simulink model "vehicle_model_June_25th_2024"  (R2022b)
settings: Solver=ode1  StartTime=0.0  StopTime=1068  FixedStep=0.01  MaxStep=0.1  RelTol=1e-3
values from neighbouring files (symbols this model uses):
  af = 2    [vehicle_load_2024.m]
  cd = 0.30    (= 0.3)    [vehicle_load_2024.m]
  crr = 0.012    [vehicle_load_2024.m]
  mg = mc+mh*np+mp    (= 1870)    [vehicle_load_2024.m]
  n = [0:dn:8000]    [electric_drive_simple.m]
  ro = 1.2041    [vehicle_load_2024.m]
  rt = 4.6    [vehicle_load_2024.m]
  rw = wd/2*25.4e-3+wt*ar/100*1e-3    (= 0.33025)    [vehicle_load_2024.m]
undefined symbols (not defined in the file or in its folder): t_roma_san_basilio, tm, vkm_roma_san_basilio
libraries: simulink x28
settings Model: Creator=claudio.rossi  LastModifiedBy=claudio.rossi
settings DebuggingCC: ParameterOverflowMsg=none  ParameterUnderflowMsg=error  ParameterPrecisionLossMsg=none

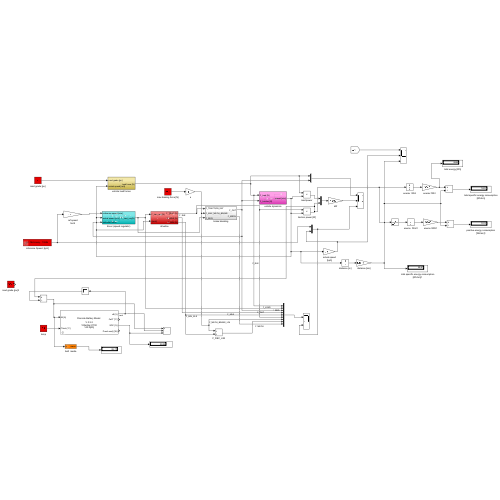
[thumbnail: Simulink's stored preview of the top-level diagram]
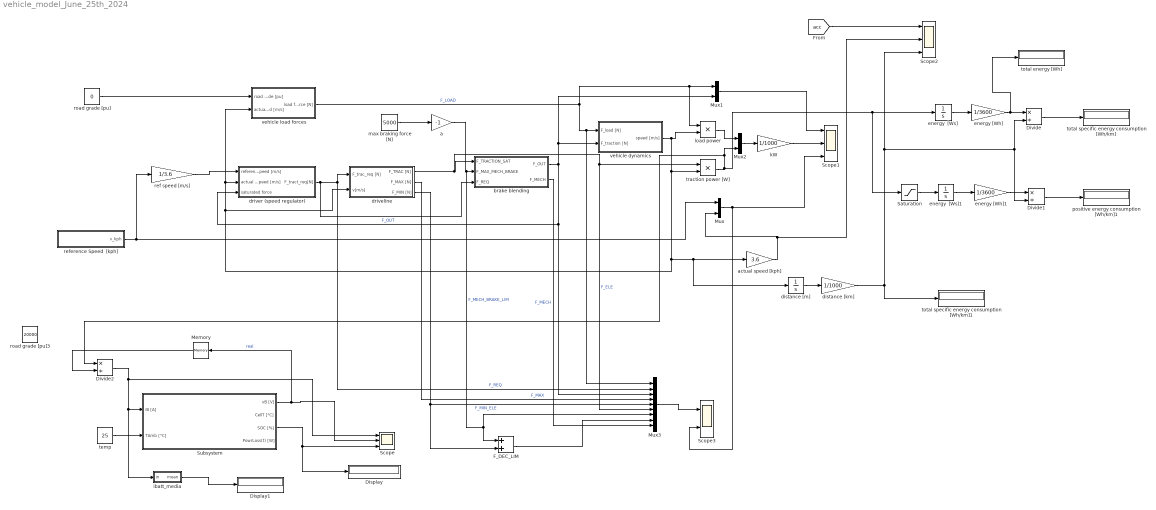
== system vehicle_model_June_25th_2024 ==
  Display : Display
  Display1 : Display
  Divide : Product  Inputs=*/
  Divide1 : Product  Inputs=*/
  Divide2 : Product  Inputs=*/
  F_DEC_LIM : Sum
  Memory : Memory  InitialCondition=400
  Mux : Mux  Inputs=2
  Mux1 : Mux  Inputs=2
  Mux2 : Mux  Inputs=2
  Mux3 : Mux  Inputs=9
  Saturation : Saturate  UpperLimit=inf  LowerLimit=0
  Scope : Scope  NumInputPorts=3
  Scope1 : Scope  NumInputPorts=3
  Scope2 : Scope  NumInputPorts=3
  Scope3 : Scope  NumInputPorts=2
  Subsystem : Subsystem  mask{seriesNumber=100, parallelNumber=28, InitialSOC=100.0, InitialSOH=100.0, BattEff=100.0, CellType=SAMSUNG	21700 	50S	5 [Ah], ThermalModelType=1D With Plastic, ThermReff=off, TRoom=20, R1Therml=2.4, R2Therml=8e-4, R3Therml=9, C1Thermal=62, C2Thermal=4.5}
      mask prompts: seriesNumber "Series Moduels Number [/]"; parallelNumber "Parallel Moduels Number [/]"; InitialSOC "Initial SoC value [%]"; InitialSOH "Initial SoH value [%]"; BattEff "Battery Efficency [%]  (Beta)"; CellType "Cell Type"; ThermalModelType "Thermal Model Type"; ThermReff "Internal Reference"; TRoom "Room Temperautre [°C]"; R1Therml "Core Resistence (R1)  [K/W]"; R2Therml "Can Resistence (R2)  [K/W]"; R3Therml "External Resistence (R3)  [K/W]"; C1Thermal "Core Capacity (C1) [J/K]"; C2Thermal "Can Capacity (C2) [J/K]"
      mask init:
      | if ~exist('batCoeffStudent', 'var')
      |     load('batCoeffStudent.mat')
      | end
      | 
      | switch CellType
      |     case 1 %'IFR18650 EC'
      |         CellNum = 3;
      |     case 2 %'NCR18650 B'
      |         CellNum = 2;
      |     case 3 % NCR18650 GA
      |         CellNum = 4;
      |     case 4 %'INR18650 S'
      |         CellNum = 10;
      |     case 5 %'INR21700 E'
      |         CellNum = 11;
      |     case 6 %'INR21700 S'
      |         CellNum = 12;
      |     case 7 %'INR18650 VTC6'
      |         CellNum = 13;
      |     case 8 %'INR21700 VTC6A'
      |         CellNum = 14;
      |     case 9 % 'INR21700 M50T'
      |         CellNum = 6;
      |     case 10 % 'INR21700 M50T'
      |         CellNum = 5;
      |     case 11 % 'INR21700 P42A'
      |         CellNum = 7;
      |     case 12 % 'INR21700 K42'
      |         CellNum = 8;
      |     case 13 % 'INR21700 K42X'
      |         CellNum = 9;
      | end
      | j = 3;
      | batFormat = batCoeff{CellNum, j};j = j + 1;
      | cellCapacity = batCoeff{CellNum, j};
      | j = 6;
      | voltLim = batCoeff{CellNum, j};j = j + 1;
      | currLim = batCoeff{CellNum, j};
      | j = 8;
      | voc = batCoeff{CellNum, j};j = j + 1;
      | dvoc = batCoeff{CellNum, j};j = j + 1;
      | Cp = batCoeff{CellNum, j};j = j + 1;
      | R0 = batCoeff{CellNum, j};j = j + 1;
      | R0T = batCoeff{CellNum, j};j = j + 1;
      | R0SOH = batCoeff{CellNum, j};j = j + 1;
      | R1 = batCoeff{CellNum, j};j = j + 1;
      | R1T = batCoeff{CellNum, j};j = j + 1;
      | tau1 = batCoeff{CellNum, j};
      mask TypeOptions CellType: OCELL	18650	EC	1.5 [Ah] | PANASONIC	18650	B	3.2 [Ah] | PANASONIC	18650	GA	3.35 [Ah] | SAMSUNG	18650 	35E	3.35 [Ah] | SAMSUNG	21700 	50E	4.9 [Ah] | SAMSUNG	21700 	50S	5 [Ah] | MURATA 	18650	VTC6	3.12 [Ah] | MURATA 	21700	VTC6A	4 [Ah] | LG	21700 	M50T	5 [Ah] | MOLICEL 	21700	M50A	5 [Ah] | MOLICEL	21700	P42A	4.2 [Ah] | KEEPPOWER	21700	K42	4.2 [Ah] | KEEPPOWER	21700	K42X	4.2 [Ah]
      mask TypeOptions ThermalModelType: Constant | 1D With Plastic | 1D No Plastic
      mask DialogControl Container13 Prompt: Pack Parameters
      mask DialogControl Container7 Prompt: Pack Configuration
      mask DialogControl Container14 Prompt: Thermal Parameters
      mask DialogControl Container6 Prompt: Room Temperature
      mask DialogControl Container15 Prompt: Thermal Parameters
      mask Display:
      | fprintf('Discrete Battery Model \n \n \n');
      | fprintf('V 0.3.2');
      | fprintf('\n\n\n %ds%dp %s \n%5.1f[Ah]', seriesNumber,parallelNumber,batFormat, cellCapacity*parallelNumber)
      | 
      | set_param(gcb,'MaskHideContents','off')
  a : Gain  Gain=-1
  actual speed [kph] : Gain  Gain=3.6
  brake blending : Subsystem
  distance [km] : Gain  Gain=1/1000
  distance [m] : Integrator  InitialCondition=0.1
  driveline : Subsystem
  driver (speed regulator) : Subsystem
  energy  [Ws] : Integrator
  energy  [Ws]1 : Integrator
  energy [Wh] : Gain  Gain=1/3600
  energy [Wh]1 : Gain  Gain=1/3600
  ibatt_media : Subsystem  mask{T=1068}
      mask prompts: T "period [s]"
  kW : Gain  Gain=1/1000
  load power : Product
  max braking force [N] : Constant  Value=5000
  positive energy consumption [Wh/km]1 : Display
  ref speed [m/s] : Gain  Gain=1/3.6
  reference Speed  [kph] : Subsystem  mask{slct=Art. Motorway - 1068s}
      mask prompts: slct "Select Cycle"
      mask help: by mtb
      mask init:
      | load('ECE_EUDC_Artemis_Bologna_Roma_WLTC_EE_bus.mat')
      mask TypeOptions slct: ECE15 - 195s | EUDC - 400s | Art. Urban - 994s | Art. Rural - 1083s | Art. Motorway - 1068s | Roma S.Basilio - 522s | BO Viali slow - 1321s | BO Viali quick - 1215s | WLTC city - 1022s | WLTC class1 - 1612s | WLTC class2 - 1800s | WLTC class3a - 1800s | WLTC class3b - 1800s | Bus line BO 27A - 3246s | Bus line BO 27B - 3058s | Bus line BO 33 - 1850s | EE Bike Cycle - 1201s | 130kph
      mask DialogControl DescGroupVar Prompt: LEMAD Speed Cycle
      mask DialogControl DescTextVar Prompt: Function that outputs the speed reference in Km/h for the desired cycle
      mask Display:
      | switch slct
      |     case 1
      |         fprintf('ECE15 - 195s');
      |     case 2
      |         fprintf('EUDC - 400s');
      |     case 3
      |         fprintf('Art. Urban - 994s');
      |     case 4
      |         fprintf('Art. Rural - 1083s');
      |     case 5
      |         fprintf('Art. Motorway - 1068s');
      |     case 6
      |         fprintf('Roma S.Basilio - 522s');
      |     case 7
      |         fprintf('BO Viali slow - 1321s');
      |     case 8
      |         fprintf('BO Viali quick - 1215s');
      |     case 9
      |         fprintf('WLTC city - 1022s');
      |     case 10
      |         fprintf('WLTC class1 - 1612s');
      |     case 11
      |         fprintf('WLTC class2 - 1800s');
      |     case 12
      |         fprintf('WLTC class3a - 1800s');
      |     case 13
      |         fprintf('WLTC class3b - 1800s');
      |     case 14
      |         fprintf('Bus line BO 27A - 3246s');
      |     case 15
      |         fprintf('Bus line BO 27A - 3058s');
      |     case 16
      |         fprintf('Bus line BO 33 - 1850s');
      |     case 17
      |         fprintf('EE Bike Cycle - 1201s');
      |     case 18
      |         fprintf('130kph');
      | end
  road grade [pu] : Constant  Value=0
  road grade [pu]3 : Constant  Value=20000
  temp : Constant  Value=25
  total energy [Wh] : Display
  total specific energy consumption [Wh/km] : Display
  total specific energy consumption [Wh/km]1 : Display
  traction power [W] : Product
  vehicle dynamics : Subsystem
  vehicle load forces : Subsystem
  wires:
  driver (speed regulator)/1(F_tract_req[N]) -> brake blending/3(F_REQ), driveline/1(F_trac_req [N]), Mux3/2  "F_REQ"
  vehicle load forces/1(load force [N]) -> load power/1, Mux1/1, Mux3/1, vehicle dynamics/1(F_load [N])  "F_LOAD"
  road grade [pu]/1 -> vehicle load forces/1(road grade [pu])
  ref speed [m/s]/1 -> driver (speed regulator)/1(reference speed [m/s])
  vehicle dynamics/1(speed [m/s]) -> load power/2, driveline/2(v[m/s]), vehicle load forces/2(actual speed [m/s]), driver (speed regulator)/2(actual speed [m/s]), distance [m]/1, actual speed [kph]/1, traction power [W]/2
  reference Speed  [kph]/1(v_kph) -> Mux/1, ref speed [m/s]/1
  actual speed [kph]/1 -> Scope2/2, Mux/2
  Mux/1 -> Scope3/2, Scope1/3
  load power/1 -> Mux2/1
  traction power [W]/1 -> Divide2/1, Mux2/2, Saturation/1, energy  [Ws]/1
  Mux2/1 -> kW/1
  Mux1/1 -> Scope1/1
  kW/1 -> Scope1/2
  [acc] -> Scope2/1
  distance [m]/1 -> distance [km]/1
  distance [km]/1 -> total specific energy consumption [Wh/km]1/1, Divide1/2, Divide/2, Scope2/3
  energy  [Ws]/1 -> energy [Wh]/1
  energy [Wh]/1 -> total energy [Wh]/1, Divide/1
  Divide/1 -> total specific energy consumption [Wh/km]/1
  Saturation/1 -> energy  [Ws]1/1
  energy  [Ws]1/1 -> energy [Wh]1/1
  energy [Wh]1/1 -> Divide1/1
  Divide1/1 -> positive energy consumption [Wh/km]1/1
  Mux3/1 -> Scope3/1
  driveline/2(F_MAX [N]) -> Mux3/4  "F_MAX"
  driveline/3(F_MIN [N]) -> F_DEC_LIM/2, Mux3/5  "F_MIN_ELE"
  brake blending/1(F_OUT) -> Mux3/3, driver (speed regulator)/3(saturated force), vehicle dynamics/2(F_traction [N]), Mux1/2  "F_OUT"
  driveline/1(F_TRAC [N]) -> traction power [W]/1, Mux3/6, brake blending/1(F_TRACTION_SAT)  "F_ELE"
  max braking force [N]/1 -> a/1
  a/1 -> F_DEC_LIM/1, Mux3/7, brake blending/2(F_MAX_MECH_BRAKE)  "F_MECH_BRAKE_LIM"
  F_DEC_LIM/1 -> Mux3/8
  brake blending/2(F_MECH) -> Mux3/9  "F_MECH"
  Subsystem/1(vB [V]) -> Memory/1, Scope/2  "real"
  Divide2/1 -> Subsystem/1(iB [A]), ibatt_media/1(in), Scope/1
  temp/1 -> Subsystem/2(TAmb [°C])
  Subsystem/3(SOC [%]) -> Display/1, Scope/3
  ibatt_media/1(mean) -> Display1/1
  Memory/1 -> Divide2/2

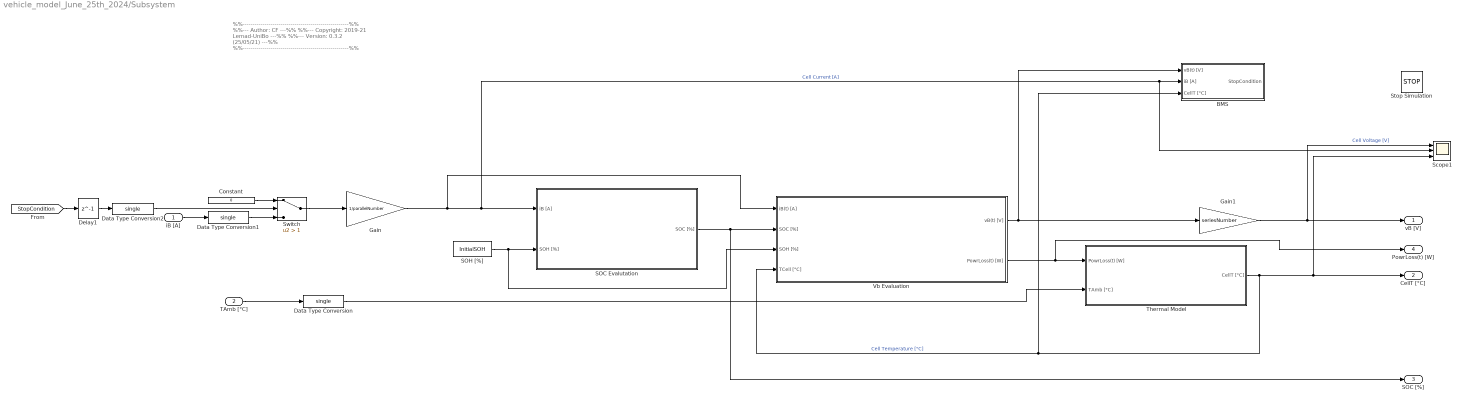
== system vehicle_model_June_25th_2024/Subsystem ==
  note: %%-----------------------------------------------------%%
      | %%--- Author: 	CF 					 ---%%
      | %%--- Copyright: 	2019-21 Lemad-UniBo ---%%
      | %%--- Version:	0.3.2 (25/05/21)		 ---%%
      | %%-----------------------------------------------------%%
  iB [A] : Inport
  TAmb [°C] : Inport  Port=2
  BMS : Subsystem
  Constant : Constant  Value=0  OutDataTypeStr=single
  Data Type Conversion : DataTypeConversion  OutDataTypeStr=single  SaturateOnIntegerOverflow=off  RndMeth=Floor
  Data Type Conversion1 : DataTypeConversion  OutDataTypeStr=single  SaturateOnIntegerOverflow=off  RndMeth=Floor
  Data Type Conversion2 : DataTypeConversion  OutDataTypeStr=single  SaturateOnIntegerOverflow=off  RndMeth=Floor
  Delay1 : Delay  DelayLength=1
  Gain : Gain  Gain=1/parallelNumber  OutDataTypeStr=single
  Gain1 : Gain  Gain=seriesNumber
  SOC Evalutation : Subsystem
      mask Display: image('SOC.PNG'); % Use "Edit Image" on toolstrip to change.
  SOH [%] : Constant  Value=InitialSOH  OutDataTypeStr=single
  Scope1 : Scope  NumInputPorts=3
  Stop Simulation : Stop
  Switch : Switch  Criteria=u2 > Threshold  Threshold=1  SaturateOnIntegerOverflow=off  InputSameDT=off
  Thermal Model : Subsystem
      mask Display: image('ThermModel.png'); % Use "Edit Image" on toolstrip to change.
  Vb Evaluation : Subsystem
      mask Display: image('SP_scheme.PNG'); % Use "Edit Image" on toolstrip to change.
  vB [V] : Outport
  CellT [°C] : Outport  Port=2
  SOC [%] : Outport  Port=3
  PowrLoss(t) [W] : Outport  Port=4
  wires:
  SOH [%]/1 -> Vb Evaluation/3(SOH [%]), SOC Evalutation/2(SOH [%])
  SOC Evalutation/1(SOC [%]) -> SOC [%]/1, Vb Evaluation/2(SOC [%])
  TAmb [°C]/1 -> Data Type Conversion/1
  Gain/1 -> SOC Evalutation/1(iB [A]), Scope1/2, BMS/2(iB [A]), Vb Evaluation/1(iB(t) [A])  "Cell Current [A]"
  Vb Evaluation/1(vB(t) [V]) -> Gain1/1, BMS/1(vB(t) [V])
  Gain1/1 -> Scope1/1, vB [V]/1  "Cell Voltage [V]"
  Vb Evaluation/2(PowrLoss(t) [W]) -> PowrLoss(t) [W]/1, Thermal Model/1(PowrLoss(t) [W])
  Thermal Model/1(CellT [°C]) -> BMS/3(CellT [°C]), Vb Evaluation/4(TCell [°C]), Scope1/3, CellT [°C]/1  "Cell Temperature [°C]"
  Switch/1 -> Gain/1
  iB [A]/1 -> Data Type Conversion1/1
  Constant/1 -> Switch/1
  Delay1/1 -> Data Type Conversion2/1
  [StopCondition] -> Delay1/1
  Data Type Conversion/1 -> Thermal Model/2(TAmb [°C])
  Data Type Conversion1/1 -> Switch/3
  Data Type Conversion2/1 -> Switch/2

== system vehicle_model_June_25th_2024/brake blending ==
  F_TRACTION_SAT : Inport
  F_MAX_MECH_BRAKE : Inport  Port=2
  F_REQ : Inport  Port=3
  Add : Sum
  Constant : Constant  Value=0
  Saturation Dynamic : simulink/Discontinuities/Saturation Dynamic  OutMin=[]  OutMax=[]  OutDataTypeStr=Inherit: Same as second input  OutDataType=fixdt(1, 16)  OutScaling=2^-10  DoSatur=off
  Subtract : Sum  Inputs=+-
  Switch : Switch  Criteria=u2 > Threshold  SaturateOnIntegerOverflow=off  InputSameDT=off
  F_OUT : Outport
  F_MECH : Outport  Port=2
  wires:
  F_TRACTION_SAT/1 -> Add/2, Subtract/2, Switch/1, Switch/2
  Switch/1 -> Subtract/1, F_OUT/1
  F_MAX_MECH_BRAKE/1 -> Add/1
  F_REQ/1 -> Saturation Dynamic/3
  Constant/1 -> Saturation Dynamic/1
  Add/1 -> Saturation Dynamic/2
  Saturation Dynamic/1 -> Switch/3
  Subtract/1 -> F_MECH/1

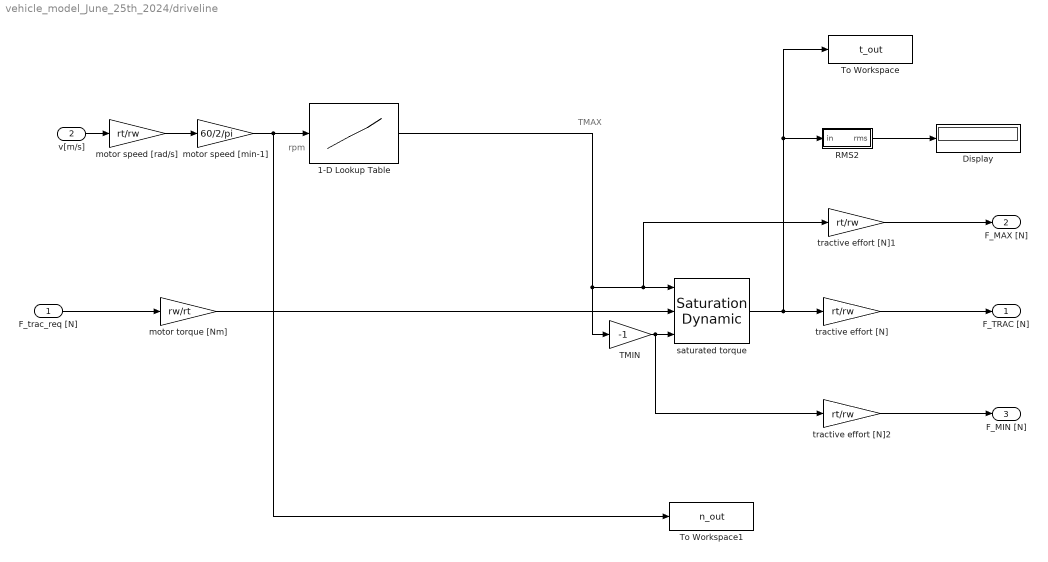
== system vehicle_model_June_25th_2024/driveline ==
  note: rpm
  note: TMAX
  F_trac_req [N] : Inport
  v[m/s] : Inport  Port=2
  1-D Lookup Table : Lookup_n-D  NumberOfTableDimensions=1  BreakpointsForDimension1=n  Table=tm  InternalRulePriority=Speed  RndMeth=Simplest
  Display : Display
  RMS2 : Subsystem  mask{T=1068}
      mask prompts: T "period [s]"
  TMIN : Gain  Gain=-1
  To Workspace : ToWorkspace  VariableName=t_out  SampleTime=-1
  To Workspace1 : ToWorkspace  VariableName=n_out  SampleTime=-1
  motor speed [min-1] : Gain  Gain=60/2/pi
  motor speed [rad/s] : Gain  Gain=rt/rw
  motor torque [Nm] : Gain  Gain=rw/rt
  saturated torque : simulink/Discontinuities/Saturation Dynamic  OutMin=[]  OutMax=[]  OutDataTypeStr=Inherit: Same as second input  OutDataType=fixdt(1, 16)  OutScaling=2^-10  DoSatur=off
  tractive effort [N] : Gain  Gain=rt/rw
  tractive effort [N]1 : Gain  Gain=rt/rw
  tractive effort [N]2 : Gain  Gain=rt/rw
  F_TRAC [N] : Outport
  F_MAX [N] : Outport  Port=2
  F_MIN [N] : Outport  Port=3
  wires:
  v[m/s]/1 -> motor speed [rad/s]/1
  motor speed [rad/s]/1 -> motor speed [min-1]/1
  motor speed [min-1]/1 -> To Workspace1/1, 1-D Lookup Table/1
  F_trac_req [N]/1 -> motor torque [Nm]/1
  1-D Lookup Table/1 -> TMIN/1, tractive effort [N]1/1, saturated torque/1
  TMIN/1 -> tractive effort [N]2/1, saturated torque/3
  motor torque [Nm]/1 -> saturated torque/2
  saturated torque/1 -> To Workspace/1, RMS2/1(in), tractive effort [N]/1
  tractive effort [N]/1 -> F_TRAC [N]/1
  tractive effort [N]1/1 -> F_MAX [N]/1
  tractive effort [N]2/1 -> F_MIN [N]/1
  RMS2/1(rms) -> Display/1

== system vehicle_model_June_25th_2024/driver (speed regulator) ==
  reference speed [m/s] : Inport
  actual speed [m/s] : Inport  Port=2
  saturated force : Inport  Port=3
  Add : Sum
  Integrator : Integrator
  KI : Gain  Gain=5000
  KP : Gain  Gain=15000
  K_desat : Gain  Gain=100
  speed error : Sum  Inputs=+-
  speed error1 : Sum  Inputs=+-
  speed error2 : Sum  Inputs=+-
  F_tract_req[N] : Outport
  wires:
  reference speed [m/s]/1 -> speed error/1
  actual speed [m/s]/1 -> speed error/2
  speed error/1 -> KI/1, KP/1
  KP/1 -> Add/1
  Integrator/1 -> Add/2
  saturated force/1 -> speed error1/2
  speed error2/1 -> Integrator/1
  KI/1 -> speed error2/1
  Add/1 -> speed error1/1, F_tract_req[N]/1
  K_desat/1 -> speed error2/2
  speed error1/1 -> K_desat/1

== system vehicle_model_June_25th_2024/ibatt_media ==
  in : Inport
  Gain1 : Gain  Gain=1/T
  Integrator : Integrator
  Subtract : Sum  Inputs=+-
  Transport Delay : TransportDelay  DelayTime=T  BufferSize=200000
  mean : Outport
  wires:
  Integrator/1 -> Subtract/1, Transport Delay/1
  in/1 -> Integrator/1
  Subtract/1 -> Gain1/1
  Transport Delay/1 -> Subtract/2
  Gain1/1 -> mean/1

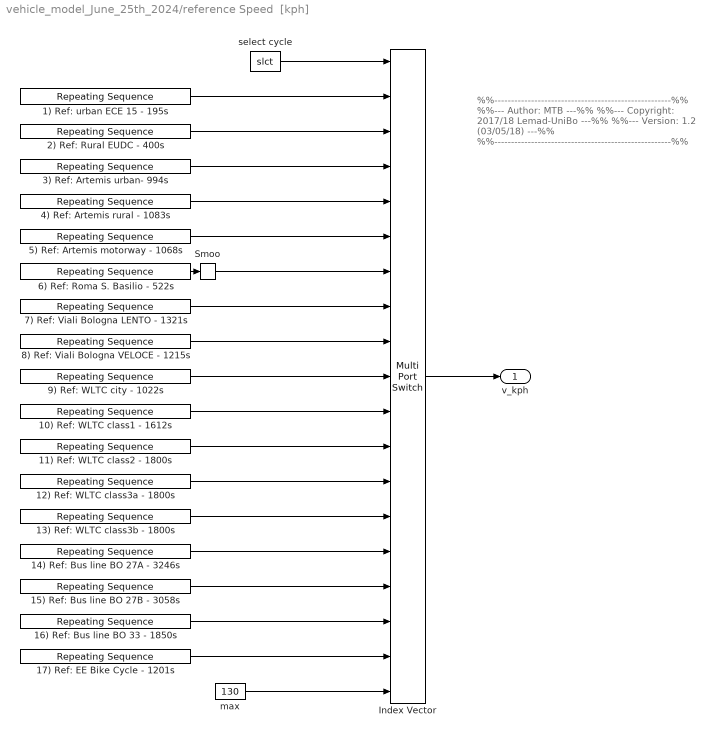
== system vehicle_model_June_25th_2024/reference Speed  [kph] ==
  note: %%-----------------------------------------------------%%
      | %%--- Author: 	MTB 				 ---%%
      | %%--- Copyright: 	2017/18 Lemad-UniBo ---%%
      | %%--- Version:	1.2 (03/05/18)		 ---%%
      | %%-----------------------------------------------------%%
  1) Ref: urban ECE 15 - 195s : simulink/Sources/Repeating Sequence  rep_seq_t=[0 11 15 23 28 49 55 61 85 96 117 123 134 143 155 163 178 188 195]  rep_seq_y=[0 0 15 15 0 0 15 15 32 32 0 0 15 35 50 50 35 35 0]
  10) Ref: WLTC class1 - 1612s : simulink/Sources/Repeating Sequence  rep_seq_t=t_wltc_class_1  rep_seq_y=vkm_wltc_class_1
  11) Ref: WLTC class2 - 1800s : simulink/Sources/Repeating Sequence  rep_seq_t=t_wltc_class_2  rep_seq_y=vkm_wltc_class_2
  12) Ref: WLTC class3a - 1800s : simulink/Sources/Repeating Sequence  rep_seq_t=t_wltc_class_3a  rep_seq_y=vkm_wltc_class_3a
  13) Ref: WLTC class3b - 1800s : simulink/Sources/Repeating Sequence  rep_seq_t=t_wltc_class_3b  rep_seq_y=vkm_wltc_class_3b
  14) Ref: Bus line BO 27A - 3246s : simulink/Sources/Repeating Sequence  rep_seq_t=t_bus_27A  rep_seq_y=vkm_bus_27A
  15) Ref: Bus line BO 27B - 3058s : simulink/Sources/Repeating Sequence  rep_seq_t=t_bus_27B  rep_seq_y=vkm_bus_27B
  16) Ref: Bus line BO 33 - 1850s : simulink/Sources/Repeating Sequence  rep_seq_t=t_bus_33  rep_seq_y=vkm_bus_33
  17) Ref: EE Bike Cycle - 1201s : simulink/Sources/Repeating Sequence  rep_seq_t=EE_time  rep_seq_y=EE_Speedkmh
  2) Ref: Rural EUDC - 400s : simulink/Sources/Repeating Sequence  rep_seq_t=t_eudc  rep_seq_y=vkm_eudc
  3) Ref: Artemis urban- 994s : simulink/Sources/Repeating Sequence  rep_seq_t=t_artemis_urban  rep_seq_y=vkm_artemis_urban
  4) Ref: Artemis rural - 1083s : simulink/Sources/Repeating Sequence  rep_seq_t=t_artemis_rural  rep_seq_y=vkm_artemis_rural
  5) Ref: Artemis motorway - 1068s : simulink/Sources/Repeating Sequence  rep_seq_t=t_artemis_motorway130  rep_seq_y=vkm_artemis_motorway130
  6) Ref: Roma S. Basilio - 522s : simulink/Sources/Repeating Sequence  rep_seq_t=[-0.1 ; t_roma_san_basilio]  rep_seq_y=[0 ; vkm_roma_san_basilio]
  7) Ref: Viali Bologna LENTO - 1321s : simulink/Sources/Repeating Sequence  rep_seq_t=t_bologna_viali_lento  rep_seq_y=vkm_bologna_viali_lento
  8) Ref: Viali Bologna VELOCE - 1215s : simulink/Sources/Repeating Sequence  rep_seq_t=t_bologna_viali_veloce  rep_seq_y=vkm_bologna_viali_veloce
  9) Ref: WLTC city - 1022s : simulink/Sources/Repeating Sequence  rep_seq_t=t_wltc_city  rep_seq_y=vkm_wltc_city
  Index Vector : MultiPortSwitch  Inputs=18  SaturateOnIntegerOverflow=off  InputSameDT=off
  Smoo : RateLimiter  RisingSlewLimit=9  FallingSlewLimit=-9  SampleTimeMode=inherited
  max : Constant  Value=130
  select cycle : Constant  Value=slct
  v_kph : Outport
  wires:
  max/1 -> Index Vector/19
  17) Ref: EE Bike Cycle - 1201s/1 -> Index Vector/18
  16) Ref: Bus line BO 33 - 1850s/1 -> Index Vector/17
  15) Ref: Bus line BO 27B - 3058s/1 -> Index Vector/16
  14) Ref: Bus line BO 27A - 3246s/1 -> Index Vector/15
  select cycle/1 -> Index Vector/1
  2) Ref: Rural EUDC - 400s/1 -> Index Vector/3
  3) Ref: Artemis urban- 994s/1 -> Index Vector/4
  4) Ref: Artemis rural - 1083s/1 -> Index Vector/5
  5) Ref: Artemis motorway - 1068s/1 -> Index Vector/6
  Smoo/1 -> Index Vector/7
  7) Ref: Viali Bologna LENTO - 1321s/1 -> Index Vector/8
  8) Ref: Viali Bologna VELOCE - 1215s/1 -> Index Vector/9
  9) Ref: WLTC city - 1022s/1 -> Index Vector/10
  10) Ref: WLTC class1 - 1612s/1 -> Index Vector/11
  11) Ref: WLTC class2 - 1800s/1 -> Index Vector/12
  12) Ref: WLTC class3a - 1800s/1 -> Index Vector/13
  13) Ref: WLTC class3b - 1800s/1 -> Index Vector/14
  Index Vector/1 -> v_kph/1
  6) Ref: Roma S. Basilio - 522s/1 -> Smoo/1
  1) Ref: urban ECE 15 - 195s/1 -> Index Vector/2

== system vehicle_model_June_25th_2024/vehicle dynamics ==
  F_load [N] : Inport
  F_traction [N] : Inport  Port=2
  Facc [N] : Sum  Inputs=+-
  Integrator : Integrator
  acceleration [m/s^2] : Gain  Gain=1/mg
  speed [m/s] : Outport
  tag scope: acc=global
  wires:
  F_traction [N]/1 -> Facc [N]/1
  F_load [N]/1 -> Facc [N]/2
  Facc [N]/1 -> acceleration [m/s^2]/1
  acceleration [m/s^2]/1 -> [acc], Integrator/1
  Integrator/1 -> speed [m/s]/1

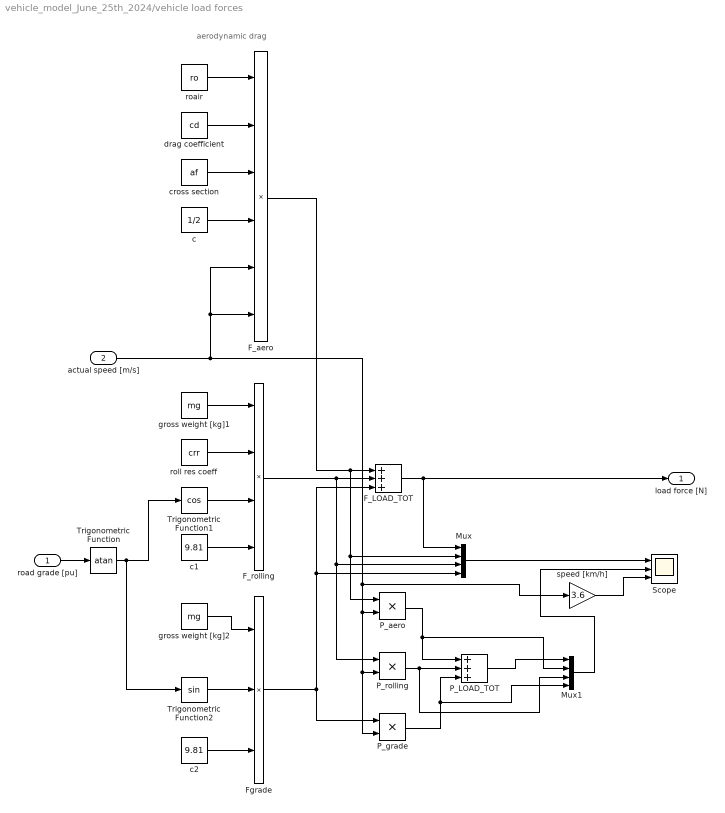
== system vehicle_model_June_25th_2024/vehicle load forces ==
  note: aerodynamic drag
  road grade [pu] : Inport
  actual speed [m/s] : Inport  Port=2
  F_LOAD_TOT : Sum  Inputs=+++
  F_aero : Product  Inputs=6
  F_rolling : Product  Inputs=4
  "Fgrade " : Product  Inputs=3
  Mux : Mux
  Mux1 : Mux
  P_LOAD_TOT : Sum  Inputs=+++
  P_aero : Product
  P_grade : Product
  P_rolling : Product
  Scope : Scope  NumInputPorts=3
  Trigonometric Function : Trigonometry  Operator=atan
  Trigonometric Function1 : Trigonometry  Operator=cos
  Trigonometric Function2 : Trigonometry
  c : Constant  Value=1/2
  c1 : Constant  Value=9.81
  c2 : Constant  Value=9.81
  "cross section " : Constant  Value=af
  drag coefficient : Constant  Value=cd
  gross weight [kg]1 : Constant  Value=mg
  gross weight [kg]2 : Constant  Value=mg
  roair : Constant  Value=ro
  roll res coeff : Constant  Value=crr
  speed [km/h] : Gain  Gain=3.6
  load force [N] : Outport
  wires:
  roair/1 -> F_aero/1
  drag coefficient/1 -> F_aero/2
  "cross section "/1 -> F_aero/3
  c/1 -> F_aero/4
  actual speed [m/s]/1 -> speed [km/h]/1, P_grade/2, P_rolling/2, P_aero/2, F_aero/5, F_aero/6
  road grade [pu]/1 -> Trigonometric Function/1
  gross weight [kg]1/1 -> F_rolling/1
  roll res coeff/1 -> F_rolling/2
  Trigonometric Function1/1 -> F_rolling/3
  c1/1 -> F_rolling/4
  gross weight [kg]2/1 -> "Fgrade "/1
  Trigonometric Function/1 -> Trigonometric Function2/1, Trigonometric Function1/1
  Trigonometric Function2/1 -> "Fgrade "/2
  c2/1 -> "Fgrade "/3
  F_aero/1 -> P_aero/1, Mux/2, F_LOAD_TOT/1
  F_rolling/1 -> P_rolling/1, Mux/3, F_LOAD_TOT/2
  "Fgrade "/1 -> Mux/4, F_LOAD_TOT/3, P_grade/1
  F_LOAD_TOT/1 -> Mux/1, load force [N]/1
  Mux/1 -> Scope/1
  P_aero/1 -> Mux1/2, P_LOAD_TOT/1
  P_rolling/1 -> Mux1/3, P_LOAD_TOT/2
  P_grade/1 -> P_LOAD_TOT/3, Mux1/4
  P_LOAD_TOT/1 -> Mux1/1
  Mux1/1 -> Scope/2
  speed [km/h]/1 -> Scope/3

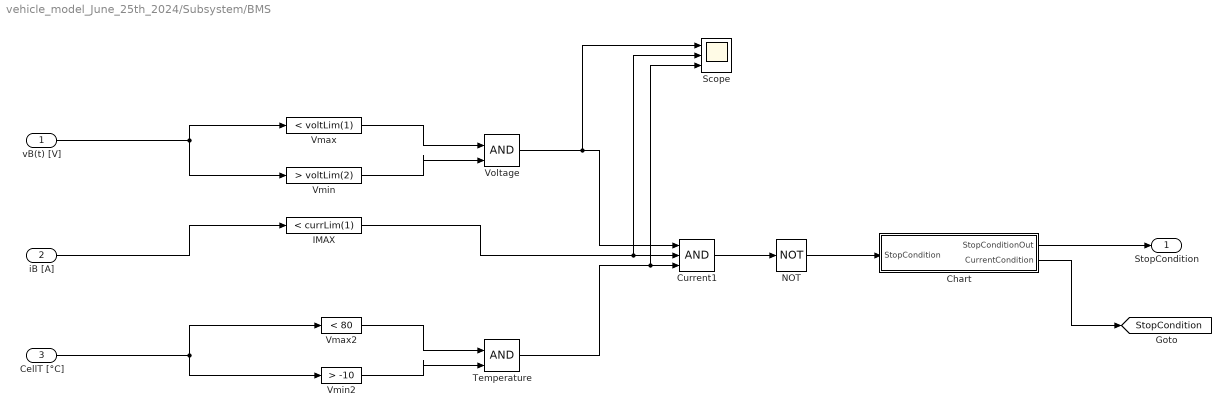
== system vehicle_model_June_25th_2024/Subsystem/BMS ==
  vB(t) [V] : Inport
  iB [A] : Inport  Port=2
  CellT [°C] : Inport  Port=3
  Chart : Stateflow chart  TreatAsAtomicUnit=on
  Current1 : Logic  Inputs=3  IconShape=distinctive  AllPortsSameDT=off  OutDataTypeStr=boolean
  IMAX : simulink/Logic and Bit Operations/Compare To Constant  relop=<  const=currLim(1)  OutDataTypeStr=boolean
  NOT : Logic  Operator=NOT  IconShape=distinctive  AllPortsSameDT=off  OutDataTypeStr=boolean
  Scope : Scope  NumInputPorts=3
  Temperature : Logic  IconShape=distinctive  AllPortsSameDT=off  OutDataTypeStr=boolean
  Vmax : simulink/Logic and Bit Operations/Compare To Constant  relop=<  const=voltLim(1)  OutDataTypeStr=boolean
  Vmax2 : simulink/Logic and Bit Operations/Compare To Constant  relop=<  const=80  OutDataTypeStr=boolean
  Vmin : simulink/Logic and Bit Operations/Compare To Constant  relop=>  const=voltLim(2)  OutDataTypeStr=boolean
  Vmin2 : simulink/Logic and Bit Operations/Compare To Constant  relop=>  const=-10  OutDataTypeStr=boolean
  Voltage : Logic  IconShape=distinctive  AllPortsSameDT=off  OutDataTypeStr=boolean
  StopCondition : Outport
  tag scope: StopCondition=global
  wires:
  Vmin/1 -> Voltage/2
  Vmax/1 -> Voltage/1
  IMAX/1 -> Scope/2, Current1/2
  Voltage/1 -> Scope/1, Current1/1
  Temperature/1 -> Scope/3, Current1/3
  Current1/1 -> NOT/1
  vB(t) [V]/1 -> Vmin/1, Vmax/1
  Vmax2/1 -> Temperature/1
  Vmin2/1 -> Temperature/2
  CellT [°C]/1 -> Vmax2/1, Vmin2/1
  iB [A]/1 -> IMAX/1
  NOT/1 -> Chart/1(StopCondition)
  Chart/2(CurrentCondition) -> [StopCondition]
  Chart/1(StopConditionOut) -> StopCondition/1

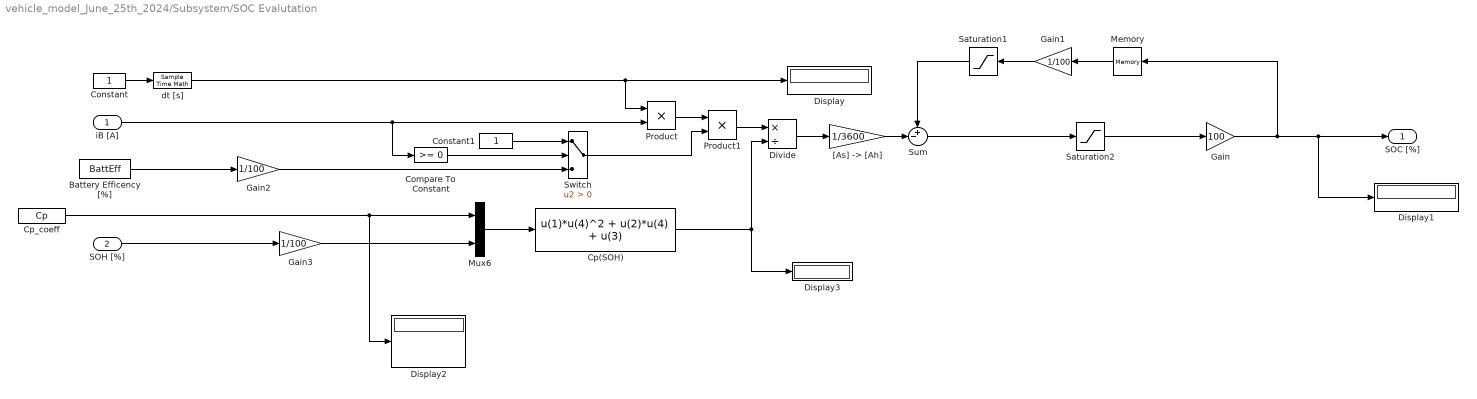
== system vehicle_model_June_25th_2024/Subsystem/SOC Evalutation ==
  iB [A] : Inport
  SOH [%] : Inport  Port=2
  Battery Efficency [%] : Constant  Value=BattEff  OutDataTypeStr=single
  Compare To Constant : simulink/Logic and Bit Operations/Compare To Constant  relop=>=  const=0  OutDataTypeStr=boolean
  Constant : Constant  OutDataTypeStr=single
  Constant1 : Constant  OutDataTypeStr=single
  Cp(SOH) : Fcn  Expr=u(1)*u(4)^2 + u(2)*u(4) + u(3)
  Cp_coeff : Constant  Value=Cp  OutDataTypeStr=single
  Display{,1..3} (4 alike) : Display
  Divide : Product  Inputs=*/
  Gain : Gain  Gain=100
  Gain1 : Gain  Gain=1/100
  Gain2 : Gain  Gain=1/100
  Gain3 : Gain  Gain=1/100
  Memory : Memory  InitialCondition=InitialSOC
  Mux6 : Mux  Inputs=2
  Product : Product  OutDataTypeStr=single
  Product1 : Product
  Saturation1 : Saturate  UpperLimit=0.999  LowerLimit=0.001
  Saturation2 : Saturate  UpperLimit=0.999  LowerLimit=0.001
  Sum : Sum  Inputs=+-|  OutDataTypeStr=single
  Switch : Switch  Criteria=u2 > Threshold  SaturateOnIntegerOverflow=off  InputSameDT=off
  "[As] -> [Ah]" : Gain  Gain=1/3600
  dt [s] : SampleTimeMath  TsampMathOp=Ts Only
  SOC [%] : Outport
  wires:
  Cp_coeff/1 -> Display2/1, Mux6/1
  Mux6/1 -> Cp(SOH)/1
  Constant/1 -> dt [s]/1
  dt [s]/1 -> Display/1, Product/1
  Cp(SOH)/1 -> Display3/1, Divide/2
  Gain/1 -> Memory/1, Display1/1, SOC [%]/1
  Saturation1/1 -> Sum/1
  Sum/1 -> Saturation2/1
  Memory/1 -> Gain1/1
  Gain1/1 -> Saturation1/1
  iB [A]/1 -> Compare To Constant/1, Product/2
  "[As] -> [Ah]"/1 -> Sum/2
  Divide/1 -> "[As] -> [Ah]"/1
  Product1/1 -> Divide/1
  Product/1 -> Product1/1
  Switch/1 -> Product1/2
  Constant1/1 -> Switch/1
  Compare To Constant/1 -> Switch/2
  Battery Efficency [%]/1 -> Gain2/1
  Gain2/1 -> Switch/3
  SOH [%]/1 -> Gain3/1
  Gain3/1 -> Mux6/2
  Saturation2/1 -> Gain/1

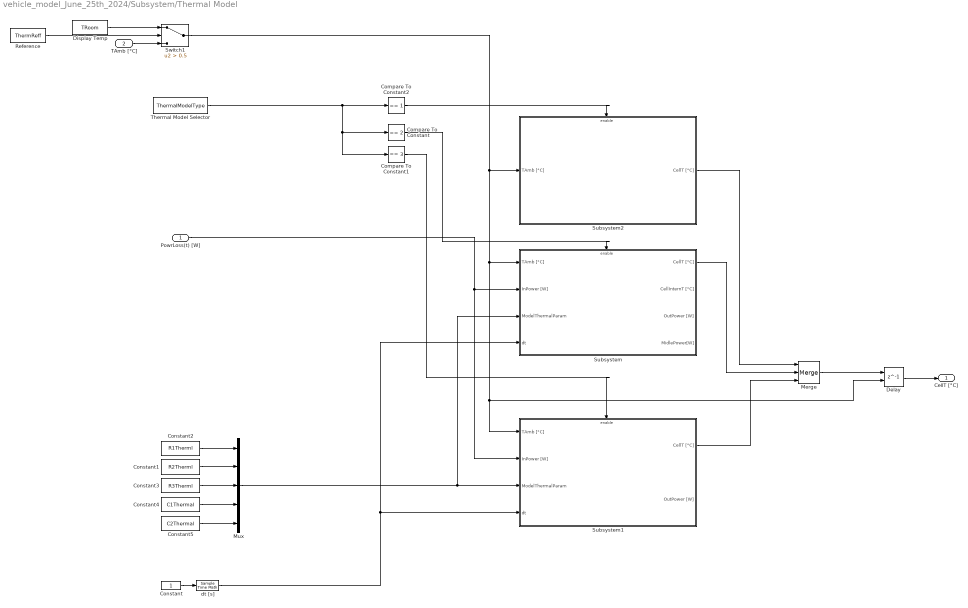
== system vehicle_model_June_25th_2024/Subsystem/Thermal Model ==
  PowrLoss(t) [W] : Inport
  TAmb [°C] : Inport  Port=2
  Compare To Constant : simulink/Logic and Bit Operations/Compare To Constant  relop===  const=2  OutDataTypeStr=boolean
  Compare To Constant1 : simulink/Logic and Bit Operations/Compare To Constant  relop===  const=3  OutDataTypeStr=boolean
  Compare To Constant2 : simulink/Logic and Bit Operations/Compare To Constant  relop===  const=1  OutDataTypeStr=boolean
  Constant : Constant  OutDataTypeStr=single
  Constant1 : Constant  Value=R2Therml  OutDataTypeStr=single
  Constant2 : Constant  Value=R1Therml  OutDataTypeStr=single
  Constant3 : Constant  Value=R3Therml  OutDataTypeStr=single
  Constant4 : Constant  Value=C1Thermal  OutDataTypeStr=single
  Constant5 : Constant  Value=C2Thermal  OutDataTypeStr=single
  Delay : Delay  DelayLength=1  InitialConditionSource=Input port
      settings: InputPortMap=u0,p4
  Display Temp : Constant  Value=TRoom  OutDataTypeStr=single
  Merge : Merge  Inputs=3
  Mux : Mux  Inputs=5
  Reference : Constant  Value=ThermReff  OutDataTypeStr=single
  Subsystem : Subsystem
  Subsystem1 : Subsystem
  Subsystem2 : Subsystem
  Switch1 : Switch  Criteria=u2 > Threshold  Threshold=0.5  SaturateOnIntegerOverflow=off  InputSameDT=off
  Thermal Model Selector : Constant  Value=ThermalModelType  OutDataTypeStr=single
  dt [s] : SampleTimeMath  TsampMathOp=Ts Only
  CellT [°C] : Outport
  wires:
  Mux/1 -> Subsystem/3(ModelThermalParam), Subsystem1/3(ModelThermalParam)
  Constant2/1 -> Mux/1
  Constant1/1 -> Mux/2
  Constant3/1 -> Mux/3
  Constant4/1 -> Mux/4
  Constant5/1 -> Mux/5
  dt [s]/1 -> Subsystem/4(dt), Subsystem1/4(dt)
  Constant/1 -> dt [s]/1
  PowrLoss(t) [W]/1 -> Subsystem1/2(InPower [W]), Subsystem/2(InPower [W])
  Thermal Model Selector/1 -> Compare To Constant/1, Compare To Constant1/1, Compare To Constant2/1
  Compare To Constant/1 -> Subsystem/Enable
  Compare To Constant1/1 -> Subsystem1/Enable
  Subsystem/1(CellT [°C]) -> Merge/2
  Subsystem1/1(CellT [°C]) -> Merge/3
  Merge/1 -> Delay/1
  Delay/1 -> CellT [°C]/1
  Display Temp/1 -> Switch1/1
  Reference/1 -> Switch1/2
  TAmb [°C]/1 -> Switch1/3
  Switch1/1 -> Subsystem2/1(TAmb [°C]), Subsystem/1(TAmb [°C]), Delay/2, Subsystem1/1(TAmb [°C])
  Compare To Constant2/1 -> Subsystem2/Enable
  Subsystem2/1(CellT [°C]) -> Merge/1

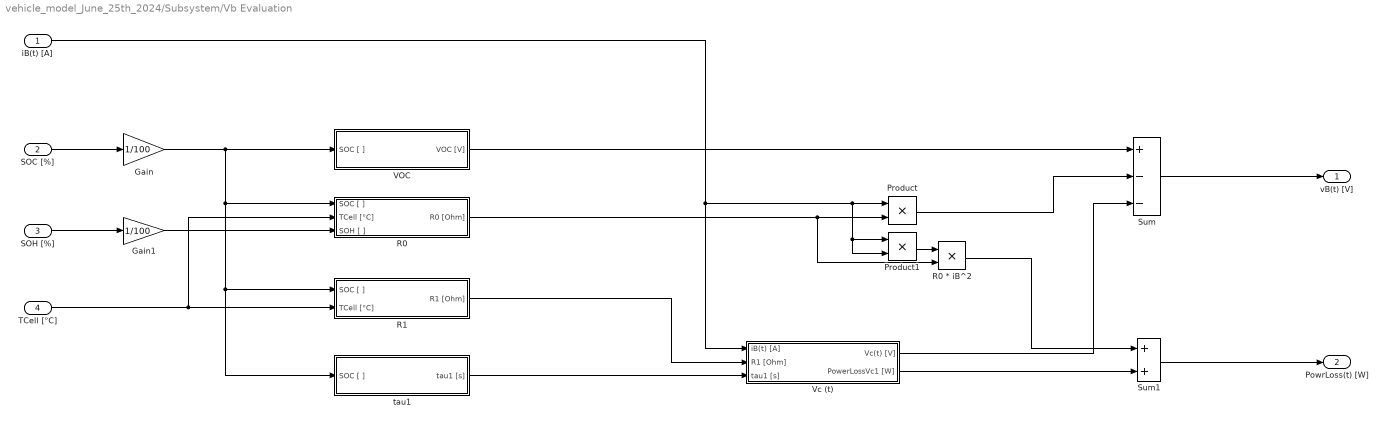
== system vehicle_model_June_25th_2024/Subsystem/Vb Evaluation ==
  iB(t) [A] : Inport
  SOC [%] : Inport  Port=2
  SOH [%] : Inport  Port=3
  TCell [°C] : Inport  Port=4
  Gain : Gain  Gain=1/100  OutDataTypeStr=single
  Gain1 : Gain  Gain=1/100
  Product : Product  OutDataTypeStr=single
  Product1 : Product  OutDataTypeStr=single
  R0 : Subsystem
  R0 * iB^2 : Product  OutDataTypeStr=single
  R1 : Subsystem
  Sum : Sum  Inputs=+--  OutDataTypeStr=single
  Sum1 : Sum  OutDataTypeStr=single
  VOC : Subsystem
  Vc (t) : Subsystem
  tau1 : Subsystem
  vB(t) [V] : Outport
  PowrLoss(t) [W] : Outport  Port=2
  wires:
  SOC [%]/1 -> Gain/1
  Gain/1 -> tau1/1(SOC [ ]), R1/1(SOC [ ]), R0/1(SOC [ ]), VOC/1(SOC [ ])
  SOH [%]/1 -> Gain1/1
  Gain1/1 -> R0/3(SOH [ ])
  TCell [°C]/1 -> R1/2(TCell [°C]), R0/2(TCell [°C])
  iB(t) [A]/1 -> Product1/2, Product1/1, Product/1, Vc (t)/1(iB(t) [A])
  R1/1(R1 [Ohm]) -> Vc (t)/2(R1 [Ohm])
  tau1/1(tau1 [s]) -> Vc (t)/3(tau1 [s])
  VOC/1(VOC [V]) -> Sum/1
  Product/1 -> Sum/2
  R0/1(R0 [Ohm]) -> R0 * iB^2/2, Product/2
  Vc (t)/1(Vc(t) [V]) -> Sum/3
  Sum/1 -> vB(t) [V]/1
  R0 * iB^2/1 -> Sum1/1
  Product1/1 -> R0 * iB^2/1
  Vc (t)/2(PowerLossVc1 [W]) -> Sum1/2
  Sum1/1 -> PowrLoss(t) [W]/1

== system vehicle_model_June_25th_2024/driveline/RMS2 ==
  note: RMS
  in : Inport
  Gain1 : Gain  Gain=1/T
  Integrator : Integrator
  Product : Product
  Sqrt : Sqrt
  Subtract : Sum  Inputs=+-
  Transport Delay : TransportDelay  DelayTime=T  BufferSize=200000
  rms : Outport
  wires:
  Gain1/1 -> Sqrt/1
  Transport Delay/1 -> Subtract/2
  Integrator/1 -> Transport Delay/1, Subtract/1
  Product/1 -> Integrator/1
  in/1 -> Product/2, Product/1
  Sqrt/1 -> rms/1
  Subtract/1 -> Gain1/1

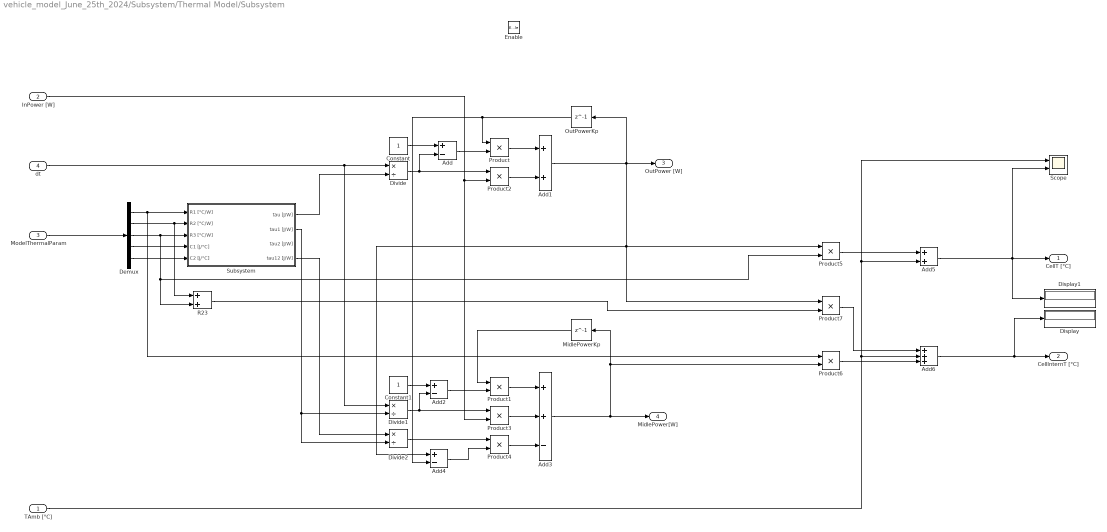
== system vehicle_model_June_25th_2024/Subsystem/Thermal Model/Subsystem ==
  TAmb [°C] : Inport
  InPower [W] : Inport  Port=2
  ModelThermalParam : Inport  Port=3
  dt : Inport  Port=4
  Enable : EnablePort
  Add : Sum  Inputs=+-
  Add1 : Sum
  Add2 : Sum  Inputs=+-
  Add3 : Sum  Inputs=++-
  Add4 : Sum  Inputs=+-
  Add5 : Sum
  Add6 : Sum  Inputs=+++
  Constant : Constant  OutDataTypeStr=single
  Constant1 : Constant  OutDataTypeStr=single
  Demux : Demux  Outputs=5
  Display : Display
  Display1 : Display
  Divide : Product  Inputs=*/
  Divide1 : Product  Inputs=*/
  Divide2 : Product  Inputs=*/
  "MidlePowerKp " : Delay  DelayLength=1
  OutPowerKp : Delay  DelayLength=1
  Product{,1..7} (8 alike) : Product  OutDataTypeStr=single
  R23 : Sum
  Scope : Scope  NumInputPorts=2
  Subsystem : Subsystem
  CellT [°C] : Outport
  CellInternT [°C] : Outport  Port=2
  OutPower [W] : Outport  Port=3
  MidlePower[W] : Outport  Port=4
  wires:
  Add6/1 -> Display/1, CellInternT [°C]/1
  Product6/1 -> Add6/3
  Product3/1 -> Add3/2
  Divide/1 -> Product2/1, Add/2
  Product5/1 -> Add5/1
  Subsystem/4(tau12 [J/W]) -> Divide2/1
  Add4/1 -> Product4/2
  Product4/1 -> Add3/3
  Add2/1 -> Product1/2
  Subsystem/1(tau [J/W]) -> Divide/2
  Product1/1 -> Add3/1
  Product/1 -> Add1/1
  Constant/1 -> Add/1
  InPower [W]/1 -> Product3/2, Product2/2
  Demux/2 -> R23/1, Subsystem/2(R2 [°C/W])
  dt/1 -> Divide1/1, Divide/1
  TAmb [°C]/1 -> Scope/1, Add5/2, Add6/2
  Demux/3 -> R23/2, Product5/2, Subsystem/3(R3 [°C/W])
  Constant1/1 -> Add2/1
  R23/1 -> Product7/2
  Divide1/1 -> Product3/1, Add2/2
  Divide2/1 -> Product4/1
  Product7/1 -> Add6/1
  Add1/1 -> OutPowerKp/1, Product7/1, Product5/1, Add4/1, OutPower [W]/1
  OutPowerKp/1 -> Add4/2, Product/1
  Demux/5 -> Subsystem/5(C2 [J/°C])
  ModelThermalParam/1 -> Demux/1
  Add/1 -> Product/2
  Demux/4 -> Subsystem/4(C1 [J/°C])
  Subsystem/2(tau1 [J/W]) -> Divide2/2, Divide1/2
  "MidlePowerKp "/1 -> Product1/1
  Product2/1 -> Add1/2
  Demux/1 -> Subsystem/1(R1 [°C/W]), Product6/1
  Add3/1 -> "MidlePowerKp "/1, Product6/2, MidlePower[W]/1
  Add5/1 -> Display1/1, Scope/2, CellT [°C]/1

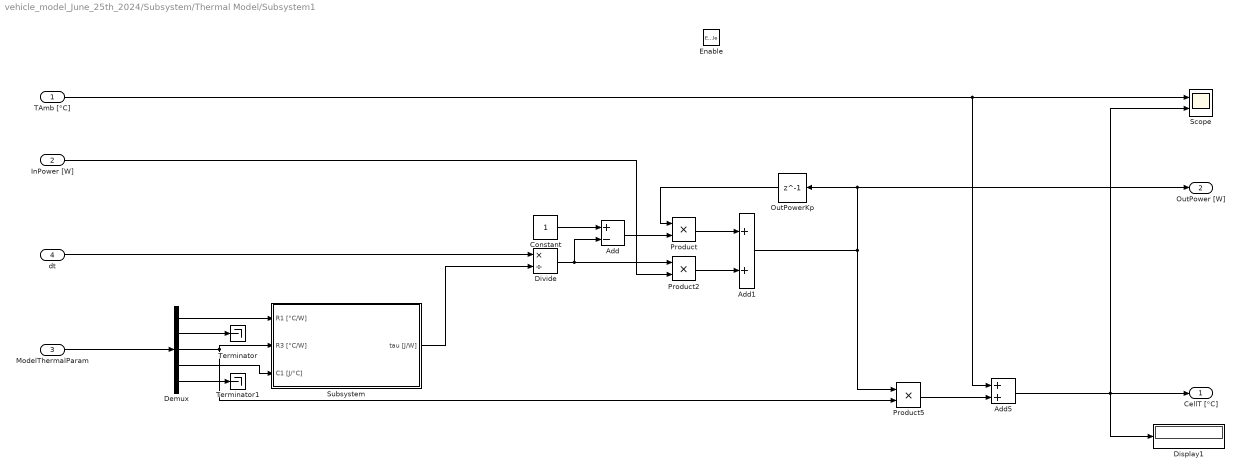
== system vehicle_model_June_25th_2024/Subsystem/Thermal Model/Subsystem1 ==
  TAmb [°C] : Inport
  InPower [W] : Inport  Port=2
  ModelThermalParam : Inport  Port=3
  dt : Inport  Port=4
  Enable : EnablePort
  Add : Sum  Inputs=+-
  Add1 : Sum
  Add5 : Sum
  Constant : Constant  OutDataTypeStr=single
  Demux : Demux  Outputs=5
  Display1 : Display
  Divide : Product  Inputs=*/
  OutPowerKp : Delay  DelayLength=1
  Product : Product  OutDataTypeStr=single
  Product2 : Product  OutDataTypeStr=single
  Product5 : Product  OutDataTypeStr=single
  Scope : Scope  NumInputPorts=2
  Subsystem : Subsystem
  Terminator : Terminator
  Terminator1 : Terminator
  CellT [°C] : Outport
  OutPower [W] : Outport  Port=2
  wires:
  Demux/1 -> Subsystem/1(R1 [°C/W])
  Demux/3 -> Product5/2, Subsystem/2(R3 [°C/W])
  dt/1 -> Divide/1
  Constant/1 -> Add/1
  Add5/1 -> Scope/2, CellT [°C]/1, Display1/1
  ModelThermalParam/1 -> Demux/1
  Divide/1 -> Product2/1, Add/2
  TAmb [°C]/1 -> Add5/1, Scope/1
  OutPowerKp/1 -> Product/1
  Product2/1 -> Add1/2
  Add1/1 -> OutPowerKp/1, OutPower [W]/1, Product5/1
  Product/1 -> Add1/1
  Subsystem/1(tau [J/W]) -> Divide/2
  InPower [W]/1 -> Product2/2
  Demux/4 -> Subsystem/3(C1 [J/°C])
  Add/1 -> Product/2
  Demux/2 -> Terminator/1
  Demux/5 -> Terminator1/1
  Product5/1 -> Add5/2

== system vehicle_model_June_25th_2024/Subsystem/Thermal Model/Subsystem2 ==
  TAmb [°C] : Inport
  Enable : EnablePort
  CellT [°C] : Outport
  wires:
  TAmb [°C]/1 -> CellT [°C]/1

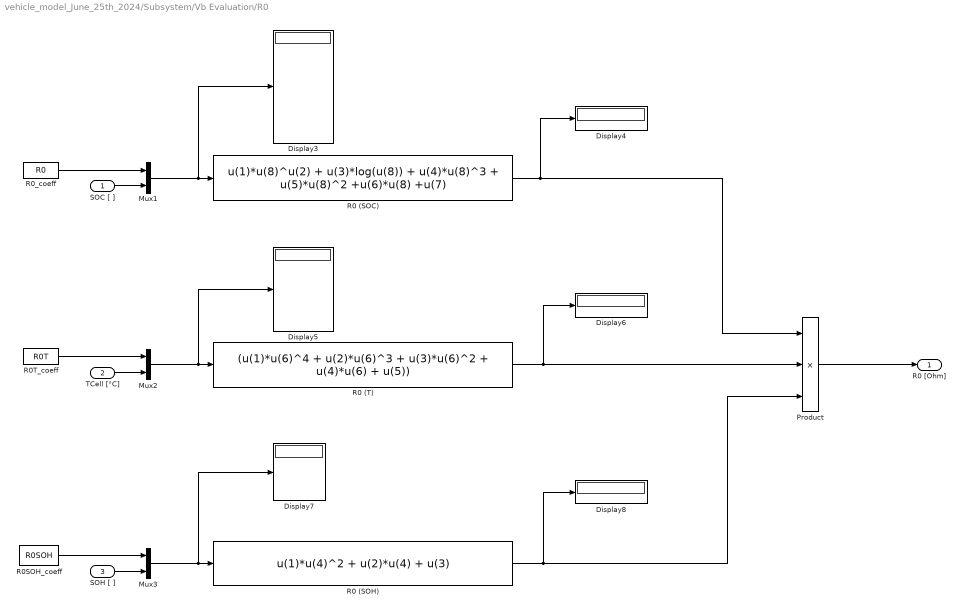
== system vehicle_model_June_25th_2024/Subsystem/Vb Evaluation/R0 ==
  SOC [ ] : Inport
  TCell [°C] : Inport  Port=2
  SOH [ ] : Inport  Port=3
  Display{3..8} (6 alike) : Display
  Mux1 : Mux  Inputs=2
  Mux2 : Mux  Inputs=2
  Mux3 : Mux  Inputs=2
  Product : Product  Inputs=3
  R0 (SOC) : Fcn  Expr=u(1)*u(8)^u(2) + u(3)*log(u(8)) + u(4)*u(8)^3 + u(5)*u(8)^2 +u(6)*u(8) +u(7)
  R0 (SOH) : Fcn  Expr=u(1)*u(4)^2 + u(2)*u(4) + u(3)
  R0 (T) : Fcn  Expr=(u(1)*u(6)^4 + u(2)*u(6)^3 + u(3)*u(6)^2 + u(4)*u(6) + u(5))
  R0SOH_coeff : Constant  Value=R0SOH  OutDataTypeStr=single
  R0T_coeff : Constant  Value=R0T  OutDataTypeStr=single
  R0_coeff : Constant  Value=R0  OutDataTypeStr=single
  R0 [Ohm] : Outport
  wires:
  R0 (SOH)/1 -> Display8/1, Product/3
  R0_coeff/1 -> Mux1/1
  R0SOH_coeff/1 -> Mux3/1
  R0 (SOC)/1 -> Product/1, Display4/1
  Mux3/1 -> R0 (SOH)/1, Display7/1
  Mux2/1 -> R0 (T)/1, Display5/1
  R0T_coeff/1 -> Mux2/1
  Mux1/1 -> Display3/1, R0 (SOC)/1
  Product/1 -> R0 [Ohm]/1
  R0 (T)/1 -> Display6/1, Product/2
  SOC [ ]/1 -> Mux1/2
  TCell [°C]/1 -> Mux2/2
  SOH [ ]/1 -> Mux3/2

== system vehicle_model_June_25th_2024/Subsystem/Vb Evaluation/R1 ==
  SOC [ ] : Inport
  TCell [°C] : Inport  Port=2
  Display{9..12} (4 alike) : Display
  Mux4 : Mux  Inputs=2
  Mux5 : Mux  Inputs=2
  Product : Product
  R1 (SOC) : Fcn  Expr=u(1)*u(8)^u(2) + u(3)*log(u(8)) + u(4)*u(8)^3 + u(5)*u(8)^2 +u(6)*u(8) +u(7)
  R1 (T) : Fcn  Expr=(u(1)*u(6)^4 + u(2)*u(6)^3 + u(3)*u(6)^2 + u(4)*u(6) + u(5))
  R1T_coeff : Constant  Value=R1T  OutDataTypeStr=single
  R1_coeff : Constant  Value=R1  OutDataTypeStr=single
  R1 [Ohm] : Outport
  wires:
  Product/1 -> R1 [Ohm]/1
  R1_coeff/1 -> Mux4/1
  R1 (T)/1 -> Display11/1, Product/2
  R1T_coeff/1 -> Mux5/1
  Mux5/1 -> Display10/1, R1 (T)/1
  Mux4/1 -> R1 (SOC)/1, Display9/1
  R1 (SOC)/1 -> Display12/1, Product/1
  TCell [°C]/1 -> Mux5/2
  SOC [ ]/1 -> Mux4/2

== system vehicle_model_June_25th_2024/Subsystem/Vb Evaluation/VOC ==
  SOC [ ] : Inport
  Mux : Mux  Inputs=2
  VOC(SOC) : Fcn  Expr=u(1) + u(2)*u(7)+u(3)*u(7)^2+ u(4)/u(7) + u(5)*log(u(7)) + u(6)*log(1-u(7))
  Voc Coeff : Constant  Value=voc  OutDataTypeStr=single
  VOC [V] : Outport
  wires:
  Mux/1 -> VOC(SOC)/1
  SOC [ ]/1 -> Mux/2
  Voc Coeff/1 -> Mux/1
  VOC(SOC)/1 -> VOC [V]/1

== system vehicle_model_June_25th_2024/Subsystem/Vb Evaluation/Vc (t) ==
  iB(t) [A] : Inport
  R1 [Ohm] : Inport  Port=2
  tau1 [s] : Inport  Port=3
  Add : Sum  Inputs=+-  AccumDataTypeStr=single  OutDataTypeStr=single
  Add1 : Sum  AccumDataTypeStr=single  OutDataTypeStr=single
  Constant : Constant  OutDataTypeStr=single
  Constant1 : Constant  OutDataTypeStr=single
  Divide : Product  Inputs=*/  OutDataTypeStr=single
  Divide1 : Product  Inputs=*/  OutDataTypeStr=single
  Memory : Memory
  Product : Product
  Product1 : Product  Inputs=3  OutDataTypeStr=single
  Product2 : Product  OutDataTypeStr=single
  dt [s] : SampleTimeMath  TsampMathOp=Ts Only
  Vc(t) [V] : Outport
  PowerLossVc1 [W] : Outport  Port=2
  wires:
  Divide/1 -> Product1/1, Add/2
  Product/1 -> Add1/1
  Add/1 -> Product/2
  Constant1/1 -> Add/1
  Memory/1 -> Product/1
  Add1/1 -> Vc(t) [V]/1, Product2/2, Product2/1, Memory/1
  Product1/1 -> Add1/2
  R1 [Ohm]/1 -> Divide1/2, Product1/2
  iB(t) [A]/1 -> Product1/3
  tau1 [s]/1 -> Divide/2
  Constant/1 -> dt [s]/1
  dt [s]/1 -> Divide/1
  Product2/1 -> Divide1/1
  Divide1/1 -> PowerLossVc1 [W]/1

== system vehicle_model_June_25th_2024/Subsystem/Vb Evaluation/tau1 ==
  SOC [ ] : Inport
  Display15 : Display
  Display16 : Display
  Mux7 : Mux  Inputs=2
  tau1(SOC) : Fcn  Expr=u(1)*u(5)^3 + u(2)*u(5)^2 + u(3)*u(5) + u(4)
  tau1_coeff : Constant  Value=tau1  OutDataTypeStr=single
  tau1 [s] : Outport
  wires:
  SOC [ ]/1 -> Mux7/2
  Mux7/1 -> tau1(SOC)/1, Display15/1
  tau1_coeff/1 -> Mux7/1
  tau1(SOC)/1 -> tau1 [s]/1, Display16/1

== system vehicle_model_June_25th_2024/Subsystem/Thermal Model/Subsystem/Subsystem ==
  R1 [°C/W] : Inport
  R2 [°C/W] : Inport  Port=2
  R3 [°C/W] : Inport  Port=3
  C1 [J/°C] : Inport  Port=4
  C2 [J/°C] : Inport  Port=5
  Sum : Sum
  Tau : Sum  Inputs=+++
  Tau1 : Product
  Tau12 : Product
  Tau2 : Product
  tau [J/W] : Outport
  tau1 [J/W] : Outport  Port=2
  tau2 [J/W] : Outport  Port=3
  tau12 [J/W] : Outport  Port=4
  wires:
  Tau1/1 -> tau1 [J/W]/1, Tau/1
  Sum/1 -> Tau12/1, Tau2/1
  Tau2/1 -> Tau/2, tau2 [J/W]/1
  C2 [J/°C]/1 -> Tau2/2
  Tau12/1 -> Tau/3, tau12 [J/W]/1
  Tau/1 -> tau [J/W]/1
  C1 [J/°C]/1 -> Tau1/2, Tau12/2
  R1 [°C/W]/1 -> Tau1/1
  R3 [°C/W]/1 -> Sum/2
  R2 [°C/W]/1 -> Sum/1

== system vehicle_model_June_25th_2024/Subsystem/Thermal Model/Subsystem1/Subsystem ==
  R1 [°C/W] : Inport
  R3 [°C/W] : Inport  Port=2
  C1 [J/°C] : Inport  Port=3
  Product : Product
  Sum : Sum
  tau [J/W] : Outport
  wires:
  R3 [°C/W]/1 -> Sum/2
  R1 [°C/W]/1 -> Sum/1
  Sum/1 -> Product/1
  C1 [J/°C]/1 -> Product/2
  Product/1 -> tau [J/W]/1

== stateflow chart vehicle_model_June_25th_2024/Subsystem/BMS/Chart ==
  state NormalState
    en:
    StopConditionOut = false;
    CurrentCondition = false;
  state Fault
    en:
    StopConditionOut = false;
    CurrentCondition = true;
    k = 0;
    during:
    k = k + 1;
    if k == 1000
    StopConditionOut = true;
    end
  (default) -> NormalState
  NormalState -> Fault : [StopCondition == 1]
  data: StopCondition input boolean; StopConditionOut output boolean; k local single; CurrentCondition output boolean
